simulink model "text00000"  (R2020b)
settings: Solver=ode15s  StartTime=0.0  StopTime=5  RelTol=1e-3
values from neighbouring files (symbols this model uses):
  A = [1  2  3  4; 5  6  7  8; 9  10  11  12]    [mytrix.mat]    (also in pisure.m = A + (-1)^(n)*(1/i))
libraries: powerlib x10, eeDiscretePi x2, powerlib_extras x1
settings Model: Creator=38061  LastModifiedBy=38061

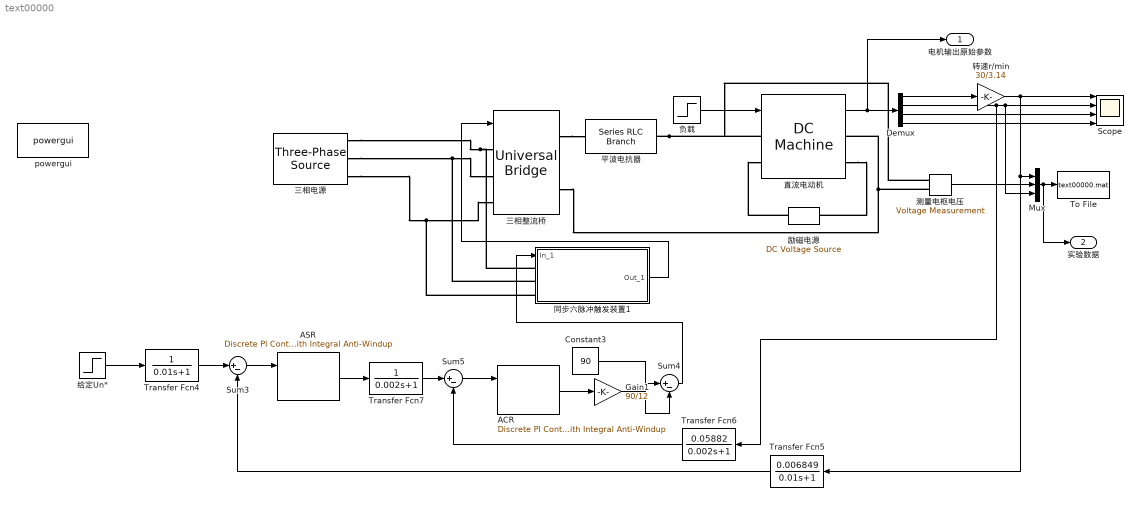
== system text00000 ==
  ACR : eeDiscretePi/Discrete PI Controller with Integral Anti-Windup  Kp=0.361846  Ki=12.0615  x0=0  B=12  A=0  Ts=50e-6
      settings: SourceProductBaseCode=PS
  ASR : eeDiscretePi/Discrete PI Controller with Integral Anti-Windup  Kp=33.50634  Ki=385.1303448  x0=0  B=12  A=0  Ts=50e-6
      settings: SourceProductBaseCode=PS
  Constant3 : Constant  Value=90
  Demux : Demux
  Gain1 : Gain  Gain=90/12
  Mux : Mux  Inputs=3
  Scope : Scope  NumInputPorts=4
  Sum3 : Sum  Inputs=|+-
  Sum4 : Sum  Inputs=|+-
  Sum5 : Sum  Inputs=|+-
  To File : ToFile  Filename=text00000.mat  SaveFormat=Timeseries
  Transfer Fcn4 : TransferFcn  Denominator=[0.01 1]
  Transfer Fcn5 : TransferFcn  Numerator=[0.006849]  Denominator=[0.01 1]
  Transfer Fcn6 : TransferFcn  Numerator=[0.05882]  Denominator=[0.002 1]
  Transfer Fcn7 : TransferFcn  Denominator=[0.002 1]
  powergui : powerlib/powergui  Priority=1  SimulationMode=Continuous  SampleTime=50e-6  frequency=60  Iterations=50  frequencyindice=50  Pbase=100e6  ErrMax=1e-4  UnitsV=kV  UnitsW=MW  buscounter=0  FunctionMessages=off  echomessages=off  EnableUseOfTLC=off  CurrentSourceSwitches=off  DisableSnubberDevices=off  DisableRonSwitches=off  DisableVfSwitches=off  DisplayEquations=off  AutomaticDiscreteSolvers=off  SolverType=Tustin/Backward Euler (TBE)  Interpol=off  ExternalGateDelay=off  methode=off  Ts=100  x0status=blocks  SPID=on  SwTol=0  HookPort=off  NonlinearTolerance=1e-4  nMaxIteration=100  ContinueOnMaxIteration=off  RestoreLinks=warning  ResistiveCurrentMeasurement=off  Frange=[0:2:500]  Ylog=off  Xlog=on  ShowGrid=off  save=off  variable=ZData  structure=0  ZoomFFT=off  StartTime=0.0  cycles=1  DisplayStyle=1  fundamental=60  FreqAxis=off  MaxFrequency=1000  frequencyindicesteady=1  RmsSteady=1  display=off
  三相整流桥 : powerlib/Power Electronics/Universal Bridge  Arms=3  SnubberResistance=1e5  SnubberCapacitance=inf  Device=Thyristors  Ron=0.5  Lon=0  ForwardVoltages="[  0  0  ]"  ForwardVoltage=0  GTOparameters=[ 10e-6 , 20e-6 ]  IGBTparameters=[ 1e-6 , 2e-6 ]  Measurements=None  Measurements_2=None  converterType=Rectifier
  三相电源 : powerlib/Electrical Sources/Three-Phase Source  InternalConnection=Yg  VoltagePhases=off  Voltage=142*sqrt(3)  PhaseAngle=0  Voltage_phases=[25e3 25e3 25e3]/sqrt(3)  PhaseAngles_phases=[0 -120 +120]  Frequency=50  NonIdealSource=on  SpecifyImpedance=off  Resistance=0.001  Inductance=0  ShortCircuitLevel=100e6  BaseVoltage=25e3  XRratio=7  BusType=swing  Pref=10e3  Qref=0  Prefabc=[10e3, 10e3, 10e3]  Qrefabc=[0, 0, 0]  Qmin=-inf  Qmax=inf
  励磁电源 : powerlib/Electrical Sources/DC Voltage Source  Amplitude=220  Measurements=None
  同步六脉冲触发装置1 : Subsystem
  平波电抗器 : powerlib/Elements/Series RLC Branch  LConnTagsString=__new0  RConnTagsString=__new0  BranchType=L  Resistance=0  Inductance=0.02  SetiL0=off  InitialCurrent=0  Capacitance=inf  Setx0=off  InitialVoltage=0  Measurements=None
  测量电枢电压 : powerlib/Measurements/Voltage Measurement  PhasorSimulation=off  OutputType=Complex  PSBequivalent=0
  直流电动机 : powerlib/Machines/DC Machine  PresetModel=No  MechanicalLoad=Torque TL  FieldType=Wound  ShowDetailedParameters=on  MeasurementBus=off  RLa="[ 0.21  0.00021]"  RLf="[ 146.7  0]"  Laf=0.84  MachineConstant=Torque constant (N.m/A)  Ke=1.8  Kt=1.8  J=0.57  Bm=0  Tf=0  w0=1  Ifinit=0.916666666666667  TsPowergui=0  TsBlock=-1
  给定Un* : Step  Time=0.5  After=10  SampleTime=0
  负载 : Step  Time=0.5  After=0  SampleTime=0
  转速r/min : Gain  Gain=30/3.14
  电机输出原始参数 : Outport
  实验数据 : Outport  Port=2
  wires:
  Mux/1 -> 实验数据/1, To File/1
  Demux/4 -> Scope/4
  转速r/min/1 -> Transfer Fcn5/1, Mux/1, Scope/1
  测量电枢电压/1 -> Mux/2
  Demux/1 -> 转速r/min/1
  Demux/3 -> Scope/3
  直流电动机/1 -> 电机输出原始参数/1, Demux/1
  Demux/2 -> Transfer Fcn6/1, Mux/3, Scope/2
  给定Un*/1 -> Transfer Fcn4/1
  Sum5/1 -> ACR/1
  ASR/1 -> Transfer Fcn7/1
  Transfer Fcn6/1 -> Sum5/2
  Transfer Fcn7/1 -> Sum5/1
  ACR/1 -> Gain1/1
  Transfer Fcn5/1 -> Sum3/2
  Gain1/1 -> Sum4/2
  Transfer Fcn4/1 -> Sum3/1
  Constant3/1 -> Sum4/1
  Sum3/1 -> ASR/1
  同步六脉冲触发装置1/1(Out_1) -> 三相整流桥/1
  Sum4/1 -> 同步六脉冲触发装置1/1(In_1)
  负载/1 -> 直流电动机/1
  connections:
  三相电源/RConn2 -- 同步六脉冲触发装置1/LConn2 -- 三相整流桥/LConn2
  三相电源/RConn1 -- 同步六脉冲触发装置1/LConn1 -- 三相整流桥/LConn1
  三相电源/RConn3 -- 同步六脉冲触发装置1/LConn3 -- 三相整流桥/LConn3
  平波电抗器/RConn1 -- 直流电动机/LConn1 -- 测量电枢电压/LConn1
  测量电枢电压/LConn2 -- 三相整流桥/RConn2 -- 直流电动机/RConn1
  三相整流桥/RConn1 -- 平波电抗器/LConn1
  励磁电源/RConn1 -- 直流电动机/LConn2
  直流电动机/RConn2 -- 励磁电源/LConn1

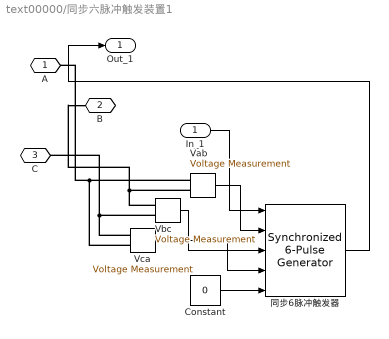
== system text00000/同步六脉冲触发装置1 ==
  In_1 : Inport
  Constant : Constant  Value=0
  Vab : powerlib/Measurements/Voltage Measurement  PhasorSimulation=off  OutputType=Complex  PSBequivalent=0
  Vbc : powerlib/Measurements/Voltage Measurement  PhasorSimulation=off  OutputType=Complex  PSBequivalent=0
  Vca : powerlib/Measurements/Voltage Measurement  PhasorSimulation=off  OutputType=Complex  PSBequivalent=0
  同步6脉冲触发器 : powerlib_extras/Control  Blocks/Synchronized 6-Pulse Generator  freq=50  pwidth=10  Double_Pulse=off
      settings: SourceProductBaseCode=PS
  A : PMIOPort  Side=Left
  B : PMIOPort  Port=2  Side=Left
  C : PMIOPort  Port=3  Side=Left
  Out_1 : Outport
  wires:
  同步6脉冲触发器/1 -> Out_1/1
  Vca/1 -> 同步6脉冲触发器/4
  Vab/1 -> 同步6脉冲触发器/2
  Constant/1 -> 同步6脉冲触发器/5
  Vbc/1 -> 同步6脉冲触发器/3
  In_1/1 -> 同步6脉冲触发器/1
  connections:
  Vca/LConn1 -- Vbc/LConn2 -- C/RConn1
  Vca/LConn2 -- Vab/LConn1 -- A/RConn1
  Vbc/LConn1 -- Vab/LConn2 -- B/RConn1
